simulink model "AnimationAttControllerVariableQuadDynamicsMdl"  (R2016b)
settings: Solver=FixedStepAuto  StartTime=0.0  StopTime=30  FixedStep=0.1  RelTol=1e-3  EnableMultiTasking=on
undefined symbols (not defined in the file): Params, QuaternionControllerAtt_Analytical, visualize_test
libraries: simulink x3
settings Model: Creator=Raj  LastModifiedBy=sailingpc
settings DataIOCC: LimitDataPoints=on  SaveFormat=Array
settings OptimizationCC: LifeSpan=inf
settings DebuggingCC: UnderspecifiedInitializationDetection=Classic  MergeDetectMultiDrivingBlocksExec=none  SolverPrmCheckMsg=warning  StateNameClashWarn=warning  SFUnexpectedBacktrackingDiag=warning  SFNoUnconditionalDefaultTransitionDiag=warning  SFExecutionAtInitializationDiag=none
settings HardwareCC: ProdBitPerPointer=32  ProdBitPerSizeT=32  ProdBitPerPtrDiffT=32  ProdLargestAtomicFloat=None  ProdIntDivRoundTo=Undefined  ProdEndianess=Unspecified  ProdWordSize=32  ProdHWDeviceType=32-bit Generic
settings ModelReferenceCC: PropagateSignalLabelsOutOfModel=off
settings GRTTargetCC: TargetLangStandard=C89/C90 (ANSI)  GeneratePreprocessorConditionals=Disable all
settings ConfigComp: CovMetricSettings=dw  CovHtmlReporting=on  CovSaveCumulativeToWorkspaceVar=on  CovSaveSingleToWorkspaceVar=on  CovExternalEMLEnable=off  CovSFcnEnable=off

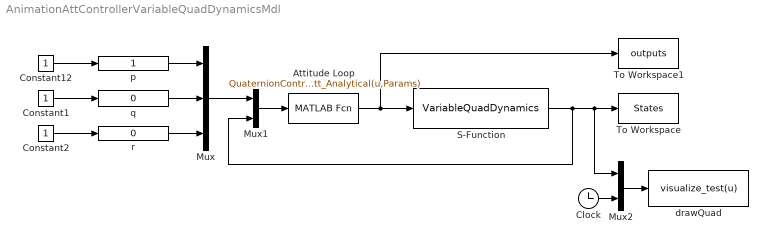
== system AnimationAttControllerVariableQuadDynamicsMdl ==
  Attitude Loop : MATLABFcn  MATLABFcn=QuaternionControllerAtt_Analytical(u,Params)  OutputDimensions=4
  Clock : Clock
  Constant1 : Constant
  Constant12 : Constant
  Constant2 : Constant
  Mux : Mux  Inputs=3
  Mux1 : Mux  Inputs=2
  Mux2 : Mux  Inputs=2
  S-Function : S-Function  FunctionName=VariableQuadDynamics  Parameters=Params  SFunctionDeploymentMode=off  EnableBusSupport=off
  To Workspace : ToWorkspace  VariableName=States  SaveFormat=Timeseries  SampleTime=-1
  To Workspace1 : ToWorkspace  VariableName=outputs  SaveFormat=Timeseries  SampleTime=-1
  drawQuad : MATLABFcn  MATLABFcn=visualize_test(u)  OutputDimensions=0
  p : simulink/Math Operations/Slider Gain  low=-20  gain=1  high=25
  q : simulink/Math Operations/Slider Gain  low=-10  gain=0  high=10
  r : simulink/Math Operations/Slider Gain  low=-10  gain=0  high=10
  wires:
  Constant12/1 -> p/1
  Constant1/1 -> q/1
  Constant2/1 -> r/1
  r/1 -> Mux/3
  q/1 -> Mux/2
  p/1 -> Mux/1
  Attitude Loop/1 -> S-Function/1, To Workspace1/1
  Mux1/1 -> Attitude Loop/1
  Mux/1 -> Mux1/1
  S-Function/1 -> Mux1/2, Mux2/1, To Workspace/1
  Mux2/1 -> drawQuad/1
  Clock/1 -> Mux2/2
